simulink model "govno"  (R2013a)
settings: Solver=ode45  StartTime=0.0  StopTime=80  RelTol=1e-3
libraries: simulink x3
settings Model: Creator=Lazaros  LastModifiedBy=Lazaros
settings DataIOCC: LimitDataPoints=off  Refine=4

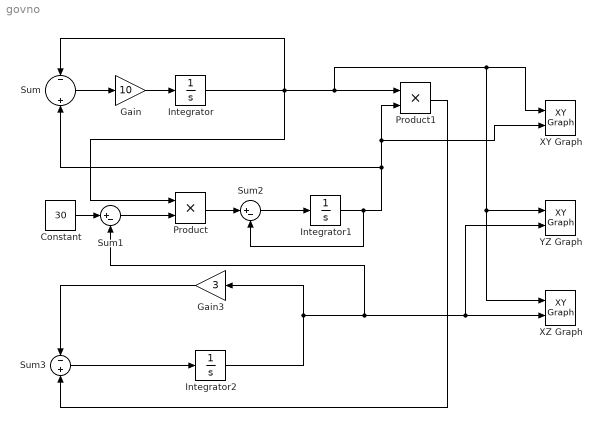
== system govno ==
  Constant : Constant  Value=30
  Gain : Gain  Gain=10
  Gain3 : Gain  Gain=3
  Integrator : Integrator  InitialCondition=5
  Integrator1 : Integrator  InitialCondition=5
  Integrator2 : Integrator  InitialCondition=5
  Product : Product
  Product1 : Product
  Sum : Sum  Inputs=-|||+
  Sum1 : Sum  Inputs=|+-
  Sum2 : Sum  Inputs=|+-
  Sum3 : Sum  Inputs=-+
  XY Graph : simulink/Sinks/XY Graph  xmin=-20  xmax=20  ymin=-30  ymax=30  st=-1
  XZ Graph : simulink/Sinks/XY Graph  xmin=-20  xmax=20  ymin=-0  ymax=60  st=-1
  YZ Graph : simulink/Sinks/XY Graph  xmin=-20  xmax=20  ymin=0  ymax=60  st=-1
  wires:
  Integrator/1 -> XZ Graph/1, YZ Graph/1, XY Graph/1, Product1/1, Product/1, Sum/1
  Sum/1 -> Gain/1
  Gain/1 -> Integrator/1
  Integrator1/1 -> Sum2/2, XY Graph/2, Product1/2, Sum/2
  Integrator2/1 -> Gain3/1, XZ Graph/2, YZ Graph/2, Sum1/2
  Sum1/1 -> Product/2
  Product/1 -> Sum2/1
  Sum2/1 -> Integrator1/1
  Sum3/1 -> Integrator2/1
  Gain3/1 -> Sum3/1
  Product1/1 -> Sum3/2
  Constant/1 -> Sum1/1
